simulink model "active_suspension"  (R2024b)
settings: Solver=VariableStepAuto  StartTime=0.0  StopTime=10.0  RelTol=1e-3
libraries: simulink x1
settings Model: Creator=anabe  LastModifiedBy=anabe

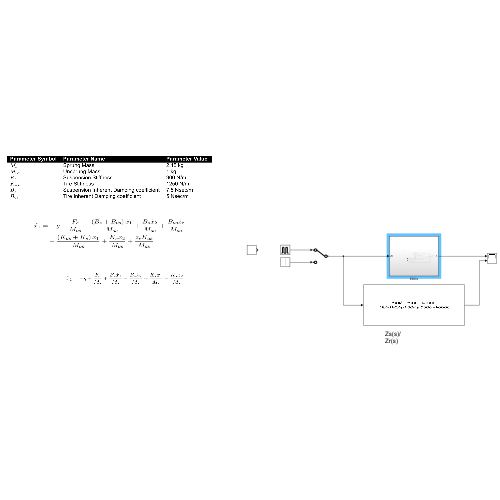
[thumbnail: Simulink's stored preview of the top-level diagram]
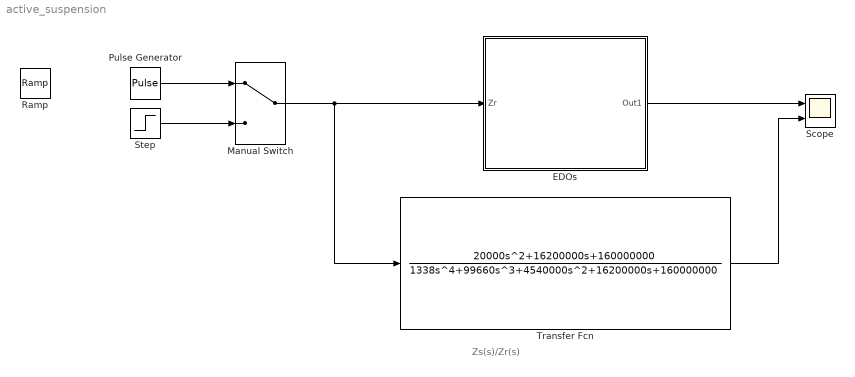
== system active_suspension ==
  note: Zs(s)/Zr(s)
  EDOs : Subsystem
  Manual Switch : ManualSwitch
  Pulse Generator : DiscretePulseGenerator  PulseType=Time based  Period=4  PulseWidth=5  PhaseDelay=1
  Ramp : simulink/Sources/Ramp  slope=1  start=0  InitialOutput=0
  Scope : Scope  NumInputPorts=2
  Step : Step  SampleTime=0
  Transfer Fcn : TransferFcn  Numerator=[20000 16200000 160000000]  Denominator=[1338 99660 4540000 16200000 160000000]
  wires:
  Manual Switch/1 -> EDOs/1(Zr), Transfer Fcn/1
  EDOs/1(Out1) -> Scope/1
  Transfer Fcn/1 -> Scope/2
  Pulse Generator/1 -> Manual Switch/1
  Step/1 -> Manual Switch/2

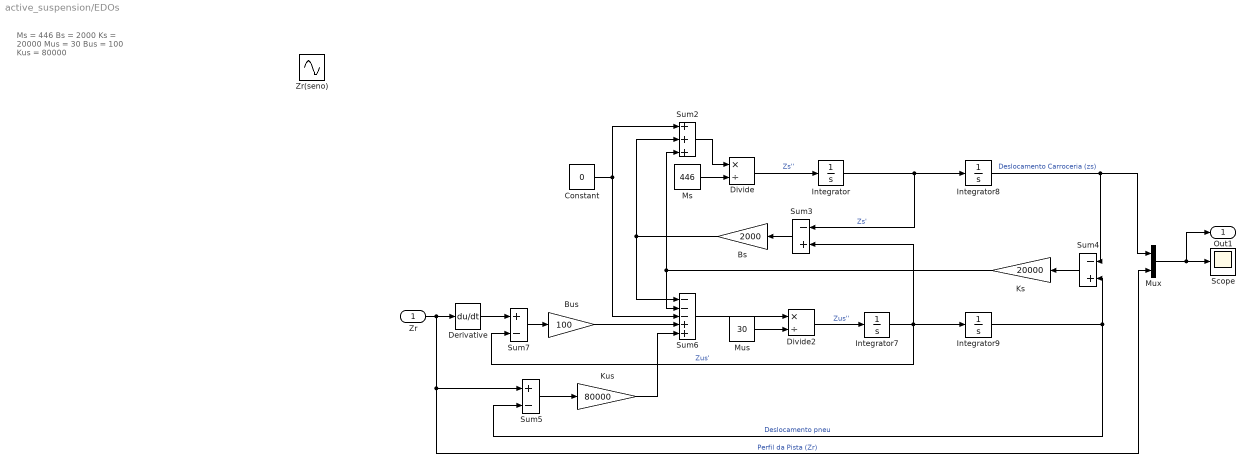
== system active_suspension/EDOs ==
  note: Ms = 446
      | Bs = 2000
      | Ks = 20000
      | Mus = 30
      | Bus = 100
      | Kus = 80000
  Zr : Inport
  Bs : Gain  Gain=2000
  Bus : Gain  Gain=100
  Constant : Constant  Value=0
  Derivative : Derivative
  Divide : Product  Inputs=*/
  Divide2 : Product  Inputs=*/
  Integrator{,7..9} (4 alike) : Integrator
  Ks : Gain  Gain=20000
  Kus : Gain  Gain=80000
  Ms : Constant  Value=446
  Mus : Constant  Value=30
  Mux : Mux  Inputs=2
  Scope : Scope
  Sum2 : Sum  Inputs=+++
  Sum3 : Sum  Inputs=-+
  Sum4 : Sum  Inputs=-+
  Sum5 : Sum  Inputs=+-
  Sum6 : Sum  Inputs=---++
  Sum7 : Sum  Inputs=+-
  Zr(seno) : Sin  Amplitude=0.5  SampleTime=0
  Out1 : Outport
  wires:
  Divide2/1 -> Integrator7/1  "Zus''"
  Bs/1 -> Sum2/2, Sum6/1
  Integrator9/1 -> Sum5/2, Sum4/2  "Deslocamento pneu"
  Sum2/1 -> Divide/1
  Sum7/1 -> Bus/1
  Sum6/1 -> Divide2/1
  Ms/1 -> Divide/2
  Bus/1 -> Sum6/4
  Integrator7/1 -> Sum7/2, Sum3/2, Integrator9/1  "Zus'"
  Sum3/1 -> Bs/1
  Sum5/1 -> Kus/1
  Ks/1 -> Sum6/2, Sum2/3
  Mus/1 -> Divide2/2
  Integrator/1 -> Integrator8/1, Sum3/1  "Zs'"
  Kus/1 -> Sum6/5
  Sum4/1 -> Ks/1
  Integrator8/1 -> Mux/1, Sum4/1  "Deslocamento Carroceria (zs)"
  Divide/1 -> Integrator/1  "Zs''"
  Derivative/1 -> Sum7/1
  Mux/1 -> Scope/1, Out1/1
  Constant/1 -> Sum2/1, Sum6/3
  Zr/1 -> Sum5/1, Mux/2, Derivative/1  "Perfil da Pista (Zr)"
